simulink library "component_lib"  (R2020b)
settings: Solver=VariableStepAuto  StartTime=0.0  StopTime=10.0  RelTol=1e-3
undefined symbols (not defined in the file or in its folder): ECCV_r, par
libraries: base_lib x70, $bdroot x59, simulink x3, pid_lib x1
(part 2 of 3)

== system component_lib/Thermal Systems ==
  note: TitanX Radiator blockset
  TH0002_radiatorCore : Subsystem  mask{HtH=1.1, StS=0.95, radmodel=52 mm}
      mask prompts: HtH "Effective header to header [m]:"; StS "Effective sideplate to sideplate [m]:"; radmodel "Core depth [m]:"
      mask init:
      | % parameter struct
      | par = struct;
      | 
      | % % get parameters
      | % par.HtH = eval(get_param(gcb, 'HtH'));
      | % par.StS = eval(get_param(gcb, 'StS'));
      | 
      | par.HtH = HtH;
      | par.StS = StS;
      | 
      | % Geometry
      | par.A_face = HtH * StS;
      | 
      | % Total heat transfer coefficient model:
      | par.cUexp = [0.7; 0.8];
      | 
      | switch radmodel
      |     
      |         case '19 mm'
      |         % Core depth
      |         par.CdT = 24e-3;
      |         
      |         % Heat trf. coefficient coefficients
      |         par.cU = [1.118075425066717e-04;
      |                   5.580064095289469e-04;
      |                   2.895685646303412e-05];
      |         
      |         % pressure drop coefficients
      |         par.c_dp_air = [37.253944105671480;
      |                          2.916659649936296e+02];         
      |         par.c_dp_clt = [19.727883408911566;
      |                          5.313528394369467];
      |         
      |         % relative area factors:
      |         rel_air = 0.752767994911226;
      |         rel_clt = 0.127946647958308;
      |     
      |     
      |         case '24 mm'
      |         % Core depth
      |         par.CdT = 24e-3;
      |         
      |         % Heat trf. coefficient coefficients
      |         par.cU = [9.815616404383520e-05;
      |                   4.676700861536502e-04;
      |                   2.415838699598361e-05];
      |         
      |         % pressure drop coefficients
      |         par.c_dp_air = [45.764851256613420;
      |                          2.404056250729179e+02];         
      |         par.c_dp_clt = [18.543378283094310;
      |                          5.151503273505832];
      |         
      |         % relative area factors:
      |         rel_air = 0.733387923444172;
      |         rel_clt = 0.132407142901122;
      |     
      |     
      |     
      |     case '42 mm'
      |         % Core depth
      |         par.CdT = 42e-3;
      |         
      |         % Heat trf. coefficient coefficients
      |         par.cU = [5.544027785616380e-05; 
      |                   2.449228920498670e-04; 
      |                   1.520415888705416e-05];
      |         
      |         % pressure drop coefficients
      |         par.c_dp_air = [36.973761781463810;
      |                          2.758340137219987e+02];
      |         par.c_dp_clt = [19.845956523612838;
      |                          5.112131585795914];
      |         
      |         % relative area factors:
      |         rel_air = 0.752767994911226;
      |         rel_clt = 0.115761252914660;
      |         
      |     case '52 mm'
      |         % Core depth
      |         par.CdT = 52e-3;
      |         
      |         % Heat trf. coefficient coefficients
      |         par.cU = [5.19516413772077e-05;
      |                   0.000198353781023090;
      |                   1.28249375163373e-05];
      |         
      |         % pressure drop coefficients
      |         par.c_dp_air = [46.462548129557995;
      |                          2.255631867184913e+02];
      |         par.c_dp_clt = [18.741626674634468;
      |                          4.871890188700768];
      |         
      |         % relative area factors:
      |         rel_air = 0.7334;
      |         rel_clt = 0.1222;
      | end
      | 
      | 
      | % Flow areas:
      | par.A_air  = rel_air * par.A_face; % Characteristic flow area
      | par.A_clt  = rel_clt * par.CdT * StS;  % Characteristic flow area
      | 
      | % fluid properties
      | setCoolantProperties;
      | setAirProperties;
      mask TypeOptions radmodel: 19 mm | 24 mm | 42 mm | 52 mm
  TH0003_coolantTank : Subsystem  mask{StS=0.95, D_con=0.055, T_0=273 + 25, radmodel=52 mm}
      mask prompts: StS "Sideplate to sideplate [m]"; D_con "Connector internal diameter [m]:"; T_0 "Temperature initial condition [K]:"; radmodel "Core depth [mm]:"
      mask init:
      | par = struct;
      | 
      | % fluid properties
      | setCoolantProperties;
      | setAirProperties;
      | 
      | % pressure drop coeffcient
      | par.zeta = 3;
      | 
      | % set core depth
      | switch radmodel
      |     
      |     case '19 mm'
      |         % Core depth
      |         par.CdT = 19e-3;
      |         
      |     case '24 mm'
      |         % Core depth
      |         par.CdT = 24e-3;
      |     
      |     case '42 mm'
      |         % Core depth
      |         par.CdT = 42e-3;
      |         
      |     case '52 mm'
      |         % Core depth
      |         par.CdT = 52e-3;
      | end
      | 
      | % Geometry
      | % tank volume
      | par.V = par.CdT.^2 * StS;
      | 
      | % inlet area
      | par.A_con = D_con.^2 .* pi/4;
      mask TypeOptions radmodel: 19 mm | 24 mm | 42 mm | 52 mm
  TH0004_radiatorPlugFlow : Subsystem  mask{HtH=1.1, StS=0.95, T_0=286, radmodel=52 mm}
      mask prompts: HtH "Header to header [m]:"; StS "Sideplate to sideplate [m]:"; T_0 "Temperature initial condition [K]:"; radmodel "Core depth [mm]:"
      mask init:
      | par = struct;
      | 
      | % get parameters
      | % par.HtH = eval(get_param(gcb, 'HtH'));
      | % par.StS = eval(get_param(gcb, 'StS'));
      | 
      | par.HtH = HtH;
      | par.StS = StS;
      | 
      | % fluid properties
      | setCoolantProperties;
      | setAirProperties;
      | 
      | 
      | % set core depth
      | switch radmodel
      |     case '42 mm'
      |         % Core depth
      |         par.CdT = 42e-3;
      |         
      |     case '52 mm'
      |         % Core depth
      |         par.CdT = 52e-3;
      | end
      mask TypeOptions radmodel: 19 mm | 24 mm | 42 mm | 52 mm
  TH0005_flowSplit : Subsystem
      mask init:
      | % fluid properties
      | setCoolantProperties;
      | setAirProperties;
  TH0006_flowConfluence : Subsystem  mask{gain=0.01}
      mask prompts: gain "Flow balance gain [-]:"
      mask init:
      | % fluid properties
      | setCoolantProperties;
      | setAirProperties;
  TH0007_airRestriction : Subsystem  mask{A=0.8, zeta=0.3}
      mask prompts: A "Area [m2]:"; zeta "Pressure drop coefficient [-]:"
      mask init:
      | % get parameters
      | % par.A    = eval(get_param(gcb, 'A'));
      | % par.zeta = eval(get_param(gcb, 'zeta'));
      | 
      | par.A    = A;
      | par.zeta = zeta;
      | 
      | % fluid properties
      | setCoolantProperties;
      | setAirProperties;
  TH0008_condenser : Subsystem  mask{HtH=0.85, StS=0.35, cdsmodel=16 mm}
      mask prompts: HtH "Header to header [m]:"; StS "Sideplate to sideplate [m]:"; cdsmodel "Core depth [m]:"
      mask init:
      | % parameter struct
      | par = struct;
      | 
      | % get parameters
      | % par.HtH = eval(get_param(gcb, 'HtH'));
      | % par.StS = eval(get_param(gcb, 'StS'));
      | 
      | par.HtH = HtH;
      | par.StS = StS;
      | 
      | 
      | switch cdsmodel
      |     case '16 mm'
      |         % Core depth
      |         par.CdT = 16-3;
      |         
      |         % pressure drop coefficients
      |         par.c_dp = [2.5; 6];
      |         
      |         
      |     case '18.8 mm'
      |         % Core depth
      |         par.CdT = 18.8e-3;
      |         
      |         % pressure drop coefficients
      |         par.c_dp = [2.7; 11];
      | end
      | 
      | % fluid properties
      | setCoolantProperties;
      | setAirProperties;
      mask TypeOptions cdsmodel: 16 mm | 18.8 mm
  TH0009_intake : Subsystem  mask{zeta=0.9}
      mask prompts: zeta "Pressure increase coefficient [-]:"
      mask init:
      | % get parameters
      | % par.zeta = eval(get_param(gcb, 'zeta'));
      | par.zeta = zeta;
      | 
      | % fluid properties
      | setCoolantProperties;
      | setAirProperties;
  TH0010_fan : Subsystem  mask{n_fan=4}
      mask prompts: n_fan "Nr. of fans [-]:"
      mask init:
      | % parameter struct
      | par = struct;
      | 
      | % get parameters
      | % par.n_fan = eval(get_param(gcb, 'n_fan'));
      | par.n_fan = n_fan;
      | 
      | 
      | % fan parameters
      | par.dpr   = -200;
      | par.q0    = 4290/3600;
      | par.dp0   = 800;
      | par.P_nom = 832;
      | 
      | 
      | % fluid properties
      | setCoolantProperties;
      | setAirProperties;
  TH0011_coolingChannel : Subsystem  mask{d=2e-3, L=50e-2, n_ch=1}
      mask prompts: d "Hydraulic diameter [m]:"; L "Length [m]:"; n_ch "Nr. of channels [-]:"
      mask init:
      | % parameter struct
      | par = struct;
      | par.d = d;
      | par.L = L;
      | 
      | % fluid properties
      | setCoolantProperties;
      | setAirProperties;
  TH0011_outletFlowBalance : Subsystem  mask{gain=0.05}
      mask prompts: gain "Dyn. balancing factor [m]:"
      mask init:
      | % fluid properties
      | setCoolantProperties;
      | setAirProperties;
  TH0011_pipe : Subsystem  mask{d=5e-2, L=1, T_0=273 + 20, p_0=2e5, W_0=2}
      mask prompts: d "Diameter [m]:"; L "Length [m]:"; T_0 "Initial temperature [K]:"; p_0 "Initial pressure [Pa]:"; W_0 "Initial flow [kg/s]:"
      mask init:
      | % parameter struct
      | par = struct;
      | 
      | % get parameters
      | % par.d = eval(get_param(gcb, 'd'));
      | % par.L = eval(get_param(gcb, 'L'));
      | 
      | par.d = d;
      | par.L = L;
      | 
      | % fluid properties
      | setCoolantProperties;
      | setAirProperties;
  TH0011_thermalMass : Subsystem  mask{m=34, cp=691, T_0=273 + 20}
      mask prompts: m "Mass [kg]:"; cp "Heat capacity [J/kgK]:"; T_0 "Initial temperature [K]:"
      mask init:
      | % fluid properties
      | setCoolantProperties;
      | setAirProperties;
  TH0012_equalSplitMerge : Subsystem  mask{n=1}
      mask prompts: n "Split/merge flow [-]"
      mask init:
      | % fluid properties
      | setCoolantProperties;
      | setAirProperties;
  TH0013_tank : Subsystem  mask{V=5e-3}
      mask prompts: V "Volume [m3]:"
      mask init:
      | % fluid properties
      | setCoolantProperties;
      | setAirProperties;
  TH0014_valve : Subsystem  mask{d=10e-2, dr=5e-2, C_d=0.9}
      mask prompts: d "Inlet port diameter [m]:"; dr "Restriction diameter [m]:"; C_d "Discharge coefficient [-]:"
      mask init:
      | % parameter struct
      | par = struct;
      | 
      | % get parameters
      | % par.d    = eval(get_param(gcb, 'd'));
      | % par.dr   = eval(get_param(gcb, 'dr'));
      | % par.C_d  = eval(get_param(gcb, 'C_d'));
      | 
      | par.d    = d;
      | par.dr   = dr;
      | par.C_d  = C_d;
      | 
      | 
      | % fluid properties
      | setCoolantProperties;
      | setAirProperties;
  TH0015_totalHeatTransfer : Subsystem
      mask init:
      | % parameter struct
      | par = struct;
      | 
      | % fluid properties
      | setCoolantProperties;
      | setAirProperties;

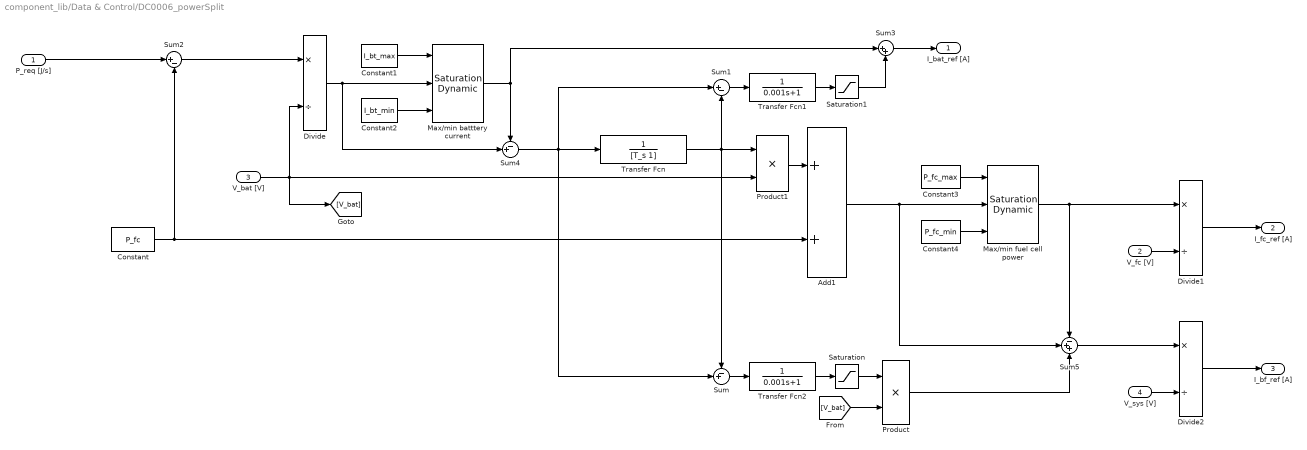
== system component_lib/Data & Control/DC0006_powerSplit ==
  P_req [J/s] : Inport
  V_fc [V] : Inport  Port=2
  V_bat [V] : Inport  Port=3
  V_sys [V] : Inport  Port=4
  Add1 : Sum
  Constant : Constant  Value=P_fc
  Constant1 : Constant  Value=I_bt_max
  Constant2 : Constant  Value=I_bt_min
  Constant3 : Constant  Value=P_fc_max
  Constant4 : Constant  Value=P_fc_min
  Divide : Product  Inputs=*/
  Divide1 : Product  Inputs=*/
  Divide2 : Product  Inputs=*/
  Max/min batttery current : simulink/Discontinuities/Saturation Dynamic  OutMin=[]  OutMax=[]  OutDataTypeStr=Inherit: Same as second input  OutDataType=fixdt(1, 16)  OutScaling=2^-10  DoSatur=off
  Max/min fuel cell power : simulink/Discontinuities/Saturation Dynamic  OutMin=[]  OutMax=[]  OutDataTypeStr=Inherit: Same as second input  OutDataType=fixdt(1, 16)  OutScaling=2^-10  DoSatur=off
  Product : Product
  Product1 : Product
  Saturation : Saturate  UpperLimit=0  LowerLimit=-inf
  Saturation1 : Saturate  UpperLimit=inf  LowerLimit=0
  Sum : Sum  Inputs=-+|
  Sum1 : Sum  Inputs=|+-
  Sum2 : Sum  Inputs=|+-
  Sum3 : Sum  Inputs=|++
  Sum4 : Sum  Inputs=-+|
  Sum5 : Sum  Inputs=-++
  Transfer Fcn : TransferFcn  Denominator=[T_s 1]
  Transfer Fcn1 : TransferFcn  Denominator=[0.001 1]
  Transfer Fcn2 : TransferFcn  Denominator=[0.001 1]
  I_bat_ref [A] : Outport
  I_fc_ref [A] : Outport  Port=2
  I_bf_ref [A] : Outport  Port=3
  wires:
  Sum2/1 -> Divide/1
  Divide1/1 -> I_fc_ref [A]/1
  V_bat [V]/1 -> Product1/2, [V_bat], Divide/2
  Constant/1 -> Sum2/2, Add1/2
  Divide/1 -> Max/min batttery current/2, Sum4/2
  Constant1/1 -> Max/min batttery current/1
  Constant2/1 -> Max/min batttery current/3
  Add1/1 -> Sum5/2, Max/min fuel cell power/2
  Constant3/1 -> Max/min fuel cell power/1
  Constant4/1 -> Max/min fuel cell power/3
  Max/min fuel cell power/1 -> Sum5/1, Divide1/1
  Sum5/1 -> Divide2/1
  V_sys [V]/1 -> Divide2/2
  Divide2/1 -> I_bf_ref [A]/1
  V_fc [V]/1 -> Divide1/2
  Product1/1 -> Add1/1
  P_req [J/s]/1 -> Sum2/1
  Max/min batttery current/1 -> Sum3/1, Sum4/1
  Sum4/1 -> Sum1/1, Sum/2, Transfer Fcn/1
  Transfer Fcn/1 -> Sum1/2, Product1/1, Sum/1
  [V_bat] -> Product/2
  Saturation/1 -> Product/1
  Product/1 -> Sum5/3
  Saturation1/1 -> Sum3/2
  Sum3/1 -> I_bat_ref [A]/1
  Sum1/1 -> Transfer Fcn1/1
  Transfer Fcn1/1 -> Saturation1/1
  Sum/1 -> Transfer Fcn2/1
  Transfer Fcn2/1 -> Saturation/1

== system component_lib/Data & Control/DC0007_cathodeFlowControl ==
  note: Oxygen flow [kg/s]
  note: Reference oxygen flow [kg/s]
  I_fc [A] : Inport
  W_ca [kg/s] : Inport  Port=2
  Cells in FC stack : Constant  Value=n_cell
  F0003_reactionFlow.m : base_lib/F0003_pukrushpan2004/F0003_reactionFlow.m  SystemSampleTime=-1  VariantActivationTime=update diagram  Latency=0  AutoFrameSizeCalculation=off
  Gain : Gain  Gain=1e5
  Gain1 : Gain  Gain=-1
  Oxygen mass fraction in dry air : Constant  Value=0.23
  Oxygen stoichiometry reference : Constant  Value=lambda_O2_ref
  PID Controller : pid_lib/PID Controller  Controller=PID  Form=Parallel  TimeDomain=Continuous-time  UseExternalTs=off  SampleTime=-1  IntegratorMethod=Forward Euler  FilterMethod=Forward Euler  ControllerParametersSource=internal  P=1  I=1  D=0  UseFilter=on  N=100  TunerSelectOption=Transfer Function Based (PID Tuner App)  InitialConditionSource=internal  InitialConditionForIntegrator=0  InitialConditionForFilter=0  DifferentiatorICPrevScaledInput=0  ExternalReset=none  TrackingMode=off  Kt=1  LimitOutput=on  SatLimitsSource=internal  UpperSaturationLimit=2e4  LowerSaturationLimit=3e3  LinearizeAsGain=on  AntiWindupMode=back-calculation  Kb=1e-1  POutMin=[]  POutMax=[]  IOutMin=[]  IOutMax=[]  DOutMin=[]  DOutMax=[]  NOutMin=[]  NOutMax=[]  SumOutMin=[]  SumOutMax=[]  SaturationOutMin=[]  SaturationOutMax=[]  PParamMin=[]  PParamMax=[]  IParamMin=[]  IParamMax=[]  DParamMin=[]  DParamMax=[]  NParamMin=[]  NParamMax=[]  KbParamMin=[]  KbParamMax=[]  KtParamMin=[]  KtParamMax=[]  KbOutMin=[]  KbOutMax=[]  KtOutMin=[]  KtOutMax=[]  IntegratorOutMin=[]  IntegratorOutMax=[]  FilterOutMin=[]  FilterOutMax=[]  SumI1OutMin=[]  SumI1OutMax=[]  SumI2OutMin=[]  SumI2OutMax=[]  SumI3OutMin=[]  SumI3OutMax=[]  SumI4OutMin=[]  SumI4OutMax=[]  SumDOutMin=[]  SumDOutMax=[]  DifferentiatorOutMin=[]  DifferentiatorOutMax=[]  FilterDiffOutCoefMin=[]  FilterDiffOutCoefMax=[]  ReciprocalOutMin=[]  ReciprocalOutMax=[]  SumDenOutMin=[]  SumDenOutMax=[]  SumNumOutMin=[]  SumNumOutMax=[]  DivideOutMin=[]  DivideOutMax=[]  UdiffTsProdOutMin=[]  UdiffTsProdOutMax=[]  NTsProdOutMin=[]  NTsProdOutMax=[]  UintegralTsProdOutMin=[]  UintegralTsProdOutMax=[]  UngainTsProdOutMin=[]  UngainTsProdOutMax=[]  IntegratorContinuousStateAttributes=''  IntegratorStateMustResolveToSignalObject=off  IntegratorRTWStateStorageClass=Auto  FilterContinuousStateAttributes=''  FilterStateMustResolveToSignalObject=off  FilterRTWStateStorageClass=Auto  ParallelPVariant=InternalParameters  IdealPVariant=Disabled  IVariant=InternalParameters  DVariant=InternalParameters  IntegratorVariant=Continuous  SatVariant=Enabled  AWVariant=BackCalculation  PCopyVariant=Disabled  TRVariant=Disabled  FdbkBlocksVariant=Forward  IdealPFdbkVariant=Disabled  SatFdbkVariant=Disabled  DerivativeFilterVariant=ContFilter  NVariant=InternalParameters  NCopyVariant=Disabled  FilterICVariant=InternalICsFilter  IntegratorICVariant=InternalICs  ExternalResetVariant=Disabled  TRSumVariant=Passthrough  SumFdbkVariant=Disabled  SumVariant=Sum_PID  TsampFilterVariant=InternalTs  TsampNgainVariant=Passthrough  TsampIntegralVariant=Passthrough  ExternalSaturationOutDataTypeStr=Inherit: Same as second input
  Product : Product  Inputs=3
  Product1 : Product
  Selector : Selector  InputPortWidth=4  IndexOptions=Index vector (dialog)  Indices=2  OutputSizes=1
  Sum : Sum  Inputs=|+-
  Terminator : Terminator
  w_cmp [rad/s] : Outport
  wires:
  F0003_reactionFlow.m/2 -> Selector/1
  Oxygen stoichiometry reference/1 -> Product/1
  Selector/1 -> Gain1/1
  Oxygen mass fraction in dry air/1 -> Product1/2
  F0003_reactionFlow.m/1 -> Terminator/1
  Gain1/1 -> Product/3
  Cells in FC stack/1 -> Product/2
  Product/1 -> Sum/1
  Product1/1 -> Sum/2
  Sum/1 -> Gain/1
  PID Controller/1 -> w_cmp [rad/s]/1
  Gain/1 -> PID Controller/1
  I_fc [A]/1 -> F0003_reactionFlow.m/1
  W_ca [kg/s]/1 -> Product1/1

== system component_lib/Data & Control/DC0010_anodeTankFlowControl ==
  note: Flow feedback - adjust +- 50%
  note: Flow feed-forward
  p [Pa] : Inport
  I_fc [A] : Inport  Port=2
  p_ref [Pa] : Inport  Port=3
  Cells in FC stack : Constant  Value=n_cell
  F0003_reactionFlow.m : base_lib/F0003_pukrushpan2004/F0003_reactionFlow.m  SystemSampleTime=-1  VariantActivationTime=update diagram  Latency=0  AutoFrameSizeCalculation=off
  Gain : Gain  Gain=1e-6
  Gain1 : Gain  Gain=-1
  Product : Product
  Product1 : Product
  Saturation : Saturate
  Selector : Selector  InputPortWidth=4  IndexOptions=Index vector (dialog)  Indices=1  OutputSizes=1
  Sum : Sum  Inputs=|+-
  Sum1 : Sum  Inputs=|++
  Terminator : Terminator
  W_H2_tank [kg/s] : Outport
  wires:
  Gain1/1 -> Product/2
  Selector/1 -> Gain1/1
  F0003_reactionFlow.m/1 -> Selector/1
  I_fc [A]/1 -> F0003_reactionFlow.m/1
  F0003_reactionFlow.m/2 -> Terminator/1
  Cells in FC stack/1 -> Product/1
  p_ref [Pa]/1 -> Sum/1
  p [Pa]/1 -> Sum/2
  Product/1 -> Sum1/1, Product1/1
  Sum1/1 -> W_H2_tank [kg/s]/1
  Sum/1 -> Gain/1
  Product1/1 -> Sum1/2
  Gain/1 -> Saturation/1
  Saturation/1 -> Product1/2

== system component_lib/Data & Control/SC0002_signalRead ==
  SigIdentifier : Inport
  tag scope: SigIdentifier=global
  wires:
  SigIdentifier/1 -> [SigIdentifier]

== system component_lib/Data & Control/SC0003_signalWrite ==
  y : Outport
  wires:
  [SigIdentifier] -> y/1

== system component_lib/Electrochemistry/EL0001_panasonicNCR18650PF ==
  note: Kelvin -> degC
  note: Power Loss
  I [A] : Inport
  T [K] : Inport  Port=2
  Abs : Abs
  Constant : Constant  Value=273.15
  Constant5 : Constant  Value=3.6e3
  Divide1 : Product  Inputs=*//
  F0001_cellCapacity.m : base_lib/F0001_panasonicCell/F0001_cellCapacity.m  SystemSampleTime=-1  VariantActivationTime=update diagram  Latency=0  AutoFrameSizeCalculation=off
      settings: SourceProductBaseCode=SL
  F0001_dynamicVoltage.m : base_lib/F0001_panasonicCell/F0001_dynamicVoltage.m  SystemSampleTime=-1  VariantActivationTime=update diagram  Latency=0  AutoFrameSizeCalculation=off
  F0001_ocvSOC.m : base_lib/F0001_panasonicCell/F0001_ocvSOC.m  SystemSampleTime=-1  VariantActivationTime=update diagram  Latency=0  AutoFrameSizeCalculation=off
      settings: SourceProductBaseCode=SL
  Gain : Gain  Gain=-1
  Integrator Limited : Integrator  InitialCondition=par.init_SOC  LimitOutput=on  UpperSaturationLimit=1  LowerSaturationLimit=0
  Integrator1 : Integrator  InitialCondition=zeros(5,1)
  Product : Product
  Product2 : Product
  Saturation : Saturate  UpperLimit=0.9  LowerLimit=0.1
  Sum : Sum  Inputs=|+-
  Sum1 : Sum  Inputs=+|-
  Sum2 : Sum  Inputs=|+-
  V [V] : Outport
  SOC [-] : Outport  Port=2
  Q_gen [J/s] : Outport  Port=3
  wires:
  F0001_dynamicVoltage.m/1 -> Integrator1/1
  Integrator1/1 -> F0001_dynamicVoltage.m/1
  T [K]/1 -> Sum2/1
  F0001_ocvSOC.m/1 -> Product/1, Sum/1
  Integrator Limited/1 -> SOC [-]/1, Saturation/1
  Sum/1 -> V [V]/1, Product2/2
  I [A]/1 -> F0001_dynamicVoltage.m/3, Gain/1, [i]
  Product/1 -> Sum1/1
  Product2/1 -> Sum1/2
  Sum1/1 -> Abs/1
  Abs/1 -> Q_gen [J/s]/1
  Constant/1 -> Sum2/2
  Sum2/1 -> F0001_dynamicVoltage.m/2, F0001_cellCapacity.m/1
  Constant5/1 -> Divide1/2
  F0001_cellCapacity.m/1 -> Divide1/3
  Gain/1 -> Divide1/1
  Divide1/1 -> Integrator Limited/1
  F0001_dynamicVoltage.m/2 -> Sum/2
  [i] -> Product2/1, Product/2
  Saturation/1 -> F0001_ocvSOC.m/1

== system component_lib/Electrochemistry/EL0003_pCell ==
  I [A] : Inport
  T [K] : Inport  Port=2
  F0002_pStackVoltage.m : base_lib/F0002_pStack/F0002_pStackVoltage.m  SystemSampleTime=-1  VariantActivationTime=update diagram  Latency=0  AutoFrameSizeCalculation=off
  F0003_reactionFlow.m : base_lib/F0003_pukrushpan2004/F0003_reactionFlow.m  SystemSampleTime=-1  VariantActivationTime=update diagram  Latency=0  AutoFrameSizeCalculation=off
  V [V] : Outport
  Q_gen [J/s] : Outport  Port=2
  W_an [kg/s] : Outport  Port=3
  W_ca [kg/s] : Outport  Port=4
  wires:
  I [A]/1 -> F0003_reactionFlow.m/1, F0002_pStackVoltage.m/1
  F0002_pStackVoltage.m/1 -> V [V]/1
  T [K]/1 -> F0002_pStackVoltage.m/2
  F0002_pStackVoltage.m/2 -> Q_gen [J/s]/1
  F0003_reactionFlow.m/1 -> W_an [kg/s]/1
  F0003_reactionFlow.m/2 -> W_ca [kg/s]/1

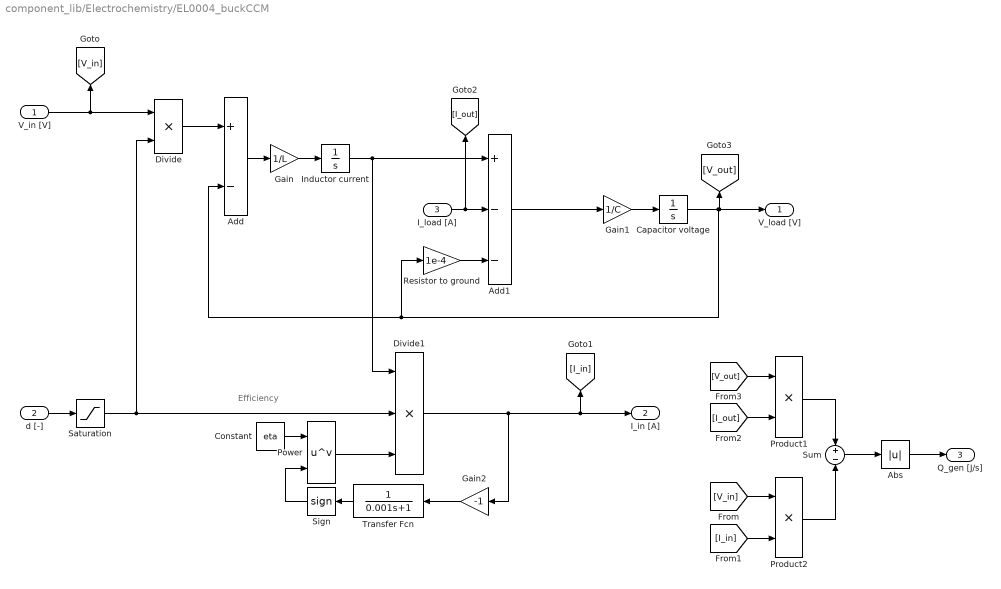
== system component_lib/Electrochemistry/EL0004_buckCCM ==
  note: Efficiency
  V_in [V] : Inport
  d [-] : Inport  Port=2
  I_load [A] : Inport  Port=3
  Abs : Abs
  Add : Sum  Inputs=+-
  Add1 : Sum  Inputs=+--
  Capacitor voltage : Integrator  InitialCondition=V_init
  Constant : Constant  Value=eta
  Divide : Product  Inputs=**
  Divide1 : Product  Inputs=***
  Gain : Gain  Gain=1/L
  Gain1 : Gain  Gain=1/C
  Gain2 : Gain  Gain=-1
  Inductor current : Integrator
  Power : Math  Operator=pow  SaturateOnIntegerOverflow=on
  Product1 : Product
  Product2 : Product
  "Resistor to ground " : Gain  Gain=1e-4
  Saturation : Saturate  UpperLimit=1  LowerLimit=0
  Sign : Signum
  Sum : Sum  Inputs=+|-
  Transfer Fcn : TransferFcn  Denominator=[0.001 1]
  V_load [V] : Outport
  I_in [A] : Outport  Port=2
  Q_gen [J/s] : Outport  Port=3
  wires:
  Divide1/1 -> Gain2/1, I_in [A]/1, [I_in]
  Abs/1 -> Q_gen [J/s]/1
  Sum/1 -> Abs/1
  Product2/1 -> Sum/2
  Product1/1 -> Sum/1
  [V_out] -> Product1/1
  [I_out] -> Product1/2
  [I_in] -> Product2/2
  [V_in] -> Product2/1
  Gain2/1 -> Transfer Fcn/1
  Transfer Fcn/1 -> Sign/1
  Constant/1 -> Power/1
  Power/1 -> Divide1/3
  Sign/1 -> Power/2
  "Resistor to ground "/1 -> Add1/3
  d [-]/1 -> Saturation/1
  V_in [V]/1 -> [V_in], Divide/1
  I_load [A]/1 -> [I_out], Add1/2
  Gain1/1 -> Capacitor voltage/1
  Add1/1 -> Gain1/1
  Inductor current/1 -> Add1/1, Divide1/1
  Gain/1 -> Inductor current/1
  Capacitor voltage/1 -> [V_out], V_load [V]/1, Add/2, "Resistor to ground "/1
  Saturation/1 -> Divide/2, Divide1/2
  Add/1 -> Gain/1
  Divide/1 -> Add/1

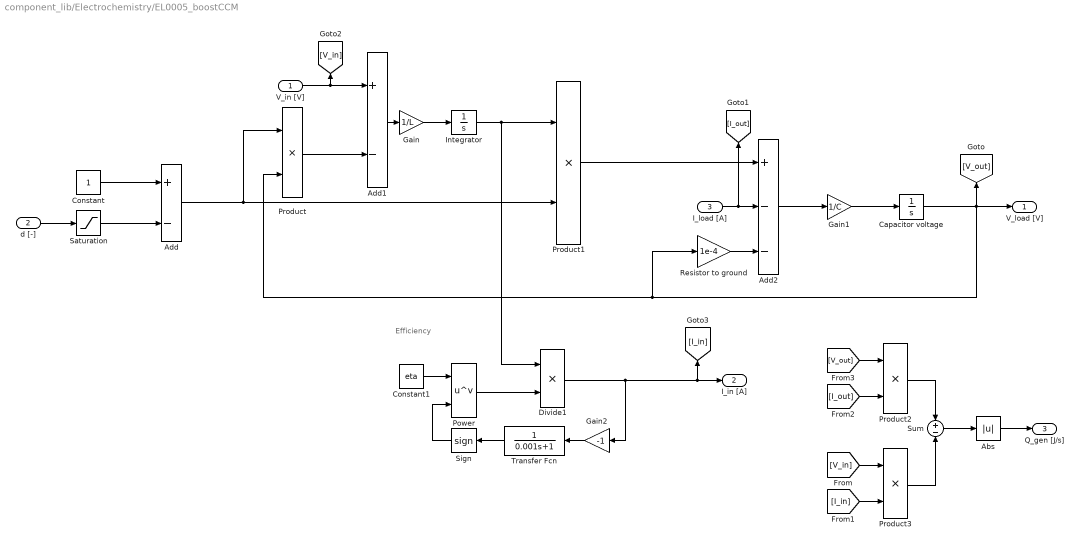
== system component_lib/Electrochemistry/EL0005_boostCCM ==
  note: Efficiency
  V_in [V] : Inport
  d [-] : Inport  Port=2
  I_load [A] : Inport  Port=3
  Abs : Abs
  Add : Sum  Inputs=+-
  Add1 : Sum  Inputs=+-
  Add2 : Sum  Inputs=+--
  Capacitor voltage : Integrator  InitialCondition=V_init
  Constant : Constant
  Constant1 : Constant  Value=eta
  Divide1 : Product  Inputs=**
  Gain : Gain  Gain=1/L
  Gain1 : Gain  Gain=1/C
  Gain2 : Gain  Gain=-1
  Integrator : Integrator
  Power : Math  Operator=pow  SaturateOnIntegerOverflow=on
  Product{,1..3} (4 alike) : Product
  Resistor to ground : Gain  Gain=1e-4
  Saturation : Saturate  UpperLimit=0.8  LowerLimit=0.2
  Sign : Signum
  Sum : Sum  Inputs=+|-
  Transfer Fcn : TransferFcn  Denominator=[0.001 1]
  V_load [V] : Outport
  I_in [A] : Outport  Port=2
  Q_gen [J/s] : Outport  Port=3
  wires:
  Divide1/1 -> I_in [A]/1, [I_in], Gain2/1
  Abs/1 -> Q_gen [J/s]/1
  Sum/1 -> Abs/1
  [V_out] -> Product2/1
  [V_in] -> Product3/1
  [I_out] -> Product2/2
  [I_in] -> Product3/2
  Product2/1 -> Sum/1
  Product3/1 -> Sum/2
  Power/1 -> Divide1/2
  Transfer Fcn/1 -> Sign/1
  Gain2/1 -> Transfer Fcn/1
  Sign/1 -> Power/2
  Constant1/1 -> Power/1
  Resistor to ground/1 -> Add2/3
  V_in [V]/1 -> Add1/1, [V_in]
  d [-]/1 -> Saturation/1
  I_load [A]/1 -> Add2/2, [I_out]
  Gain1/1 -> Capacitor voltage/1
  Add2/1 -> Gain1/1
  Product1/1 -> Add2/1
  Integrator/1 -> Product1/1, Divide1/1
  Add1/1 -> Gain/1
  Product/1 -> Add1/2
  Add/1 -> Product1/2, Product/1
  Gain/1 -> Integrator/1
  Capacitor voltage/1 -> V_load [V]/1, [V_out], Product/2, Resistor to ground/1
  Constant/1 -> Add/1
  Saturation/1 -> Add/2

== system component_lib/Electrochemistry/EL0006_parallelVoltageSources ==
  V_1 [V] : Inport
  I_load [A] : Inport  Port=2
  V_2 [V] : Inport  Port=3
  Divide : Product  Inputs=*/
  Divide1 : Product  Inputs=*/
  Gain : Gain  Gain=1/C
  Gain1 : Gain  Gain=1e-3
  R : Constant  Value=R
  Sum : Sum  Inputs=|+-
  Sum1 : Sum  Inputs=-+|
  Sum2 : Sum  Inputs=|+-
  Sum3 : Sum  Inputs=+-+
  V_4 : Integrator  InitialCondition=V_init
  I_1 [A] : Outport
  V_3 [V] : Outport  Port=2
  I_2 [A] : Outport  Port=3
  wires:
  Gain1/1 -> Sum/2
  Sum/1 -> Gain/1
  Sum3/1 -> Sum/1
  V_4/1 -> Sum1/1, Gain1/1, Sum2/2, V_3 [V]/1
  Divide1/1 -> Sum3/3, I_2 [A]/1
  V_1 [V]/1 -> Sum1/2
  I_load [A]/1 -> Sum3/2
  Gain/1 -> V_4/1
  Divide/1 -> Sum3/1, I_1 [A]/1
  V_2 [V]/1 -> Sum2/1
  Sum2/1 -> Divide1/1
  R/1 -> Divide/2, Divide1/2
  Sum1/1 -> Divide/1

== system component_lib/Gas Exchange/GE0001_humidGasSupply ==
  Constant : Constant  Value=par.p_tot
  Constant1 : Constant  Value=par.RH
  Constant2 : Constant  Value=par.T
  Constant3 : Constant  Value=par.x_H2
  Constant4 : Constant  Value=par.x_O2
  F0010_pressureSupply.m : base_lib/F0010_gasFlow/F0010_pressureSupply.m  SystemSampleTime=-1  VariantActivationTime=update diagram  Latency=0  AutoFrameSizeCalculation=off
  F0010_vaporSaturationPressure.m : base_lib/F0010_gasFlow/F0010_vaporSaturationPressure.m  SystemSampleTime=-1  VariantActivationTime=update diagram  Latency=0  AutoFrameSizeCalculation=off
  p (p x 4) : Outport
  T [K] : Outport  Port=2
  wires:
  Constant2/1 -> T [K]/1, F0010_vaporSaturationPressure.m/1
  Constant/1 -> F0010_pressureSupply.m/1
  F0010_vaporSaturationPressure.m/1 -> F0010_pressureSupply.m/5
  Constant1/1 -> F0010_pressureSupply.m/4
  Constant3/1 -> F0010_pressureSupply.m/2
  Constant4/1 -> F0010_pressureSupply.m/3
  F0010_pressureSupply.m/1 -> p (p x 4)/1

== system component_lib/Gas Exchange/GE0002_dynHumidGasSupply ==
  T [K] : Inport
  p_ref [Pa] : Inport  Port=2
  RH [-] : Inport  Port=3
  Constant : Constant  Value=x_H2_dry
  Constant1 : Constant  Value=x_O2_dry
  F0010_pressureSupply.m : base_lib/F0010_gasFlow/F0010_pressureSupply.m  SystemSampleTime=-1  VariantActivationTime=update diagram  Latency=0  AutoFrameSizeCalculation=off
      settings: SourceProductBaseCode=SL
  F0010_vaporSaturationPressure.m : base_lib/F0010_gasFlow/F0010_vaporSaturationPressure.m  SystemSampleTime=-1  VariantActivationTime=update diagram  Latency=0  AutoFrameSizeCalculation=off
      settings: SourceProductBaseCode=SL
  p (p x 4) : Outport
  T_out [K] : Outport  Port=2
  wires:
  p_ref [Pa]/1 -> F0010_pressureSupply.m/1
  T [K]/1 -> F0010_vaporSaturationPressure.m/1, T_out [K]/1
  F0010_vaporSaturationPressure.m/1 -> F0010_pressureSupply.m/5
  RH [-]/1 -> F0010_pressureSupply.m/4
  F0010_pressureSupply.m/1 -> p (p x 4)/1
  Constant/1 -> F0010_pressureSupply.m/2
  Constant1/1 -> F0010_pressureSupply.m/3

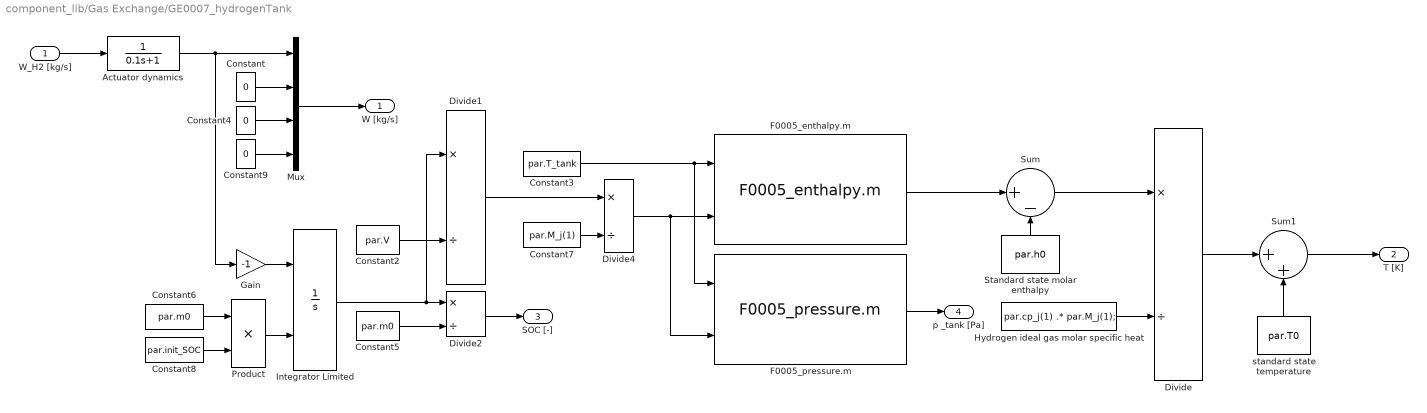
== system component_lib/Gas Exchange/GE0007_hydrogenTank ==
  W_H2 [kg/s] : Inport
  Actuator dynamics : TransferFcn  Denominator=[0.1 1]
  Constant : Constant  Value=0
  Constant2 : Constant  Value=par.V
  Constant3 : Constant  Value=par.T_tank
  Constant4 : Constant  Value=0
  Constant5 : Constant  Value=par.m0
  Constant6 : Constant  Value=par.m0
  Constant7 : Constant  Value=par.M_j(1)
  Constant8 : Constant  Value=par.init_SOC
  Constant9 : Constant  Value=0
  Divide{,1..2,4} (4 alike) : Product  Inputs=*/
  F0005_enthalpy.m : base_lib/F0005_h2Thermodynamics/F0005_enthalpy.m  SystemSampleTime=-1  VariantActivationTime=update diagram  Latency=0  AutoFrameSizeCalculation=off
  F0005_pressure.m : base_lib/F0005_h2Thermodynamics/F0005_pressure.m  SystemSampleTime=-1  VariantActivationTime=update diagram  Latency=0  AutoFrameSizeCalculation=off
  Gain : Gain  Gain=-1
  Hydrogen ideal gas molar specific heat : Constant  Value=par.cp_j(1) .* par.M_j(1);
  Integrator Limited : Integrator  InitialConditionSource=external  LimitOutput=on  LowerSaturationLimit=0
  Mux : Mux
  Product : Product
  Standard state molar enthalpy : Constant  Value=par.h0
  Sum : Sum  Inputs=|+-
  Sum1 : Sum  Inputs=|++
  standard state temperature : Constant  Value=par.T0
  W [kg/s] : Outport
  T [K] : Outport  Port=2
  SOC [-] : Outport  Port=3
  p _tank [Pa] : Outport  Port=4
  wires:
  Integrator Limited/1 -> Divide1/1, Divide2/1
  Constant2/1 -> Divide1/2
  Constant3/1 -> F0005_pressure.m/1, F0005_enthalpy.m/1
  F0005_pressure.m/1 -> p _tank [Pa]/1
  Divide2/1 -> SOC [-]/1
  Hydrogen ideal gas molar specific heat/1 -> Divide/2
  Divide1/1 -> Divide4/1
  Constant7/1 -> Divide4/2
  Divide4/1 -> F0005_enthalpy.m/2, F0005_pressure.m/2
  F0005_enthalpy.m/1 -> Sum/1
  Standard state molar enthalpy/1 -> Sum/2
  Sum/1 -> Divide/1
  Divide/1 -> Sum1/1
  standard state temperature/1 -> Sum1/2
  Sum1/1 -> T [K]/1
  Constant5/1 -> Divide2/2
  Constant6/1 -> Product/1
  Product/1 -> Integrator Limited/2
  Constant8/1 -> Product/2
  Constant9/1 -> Mux/4
  Constant/1 -> Mux/2
  Constant4/1 -> Mux/3
  Actuator dynamics/1 -> Gain/1, Mux/1
  Mux/1 -> W [kg/s]/1
  Gain/1 -> Integrator Limited/1
  W_H2 [kg/s]/1 -> Actuator dynamics/1

== system component_lib/Gas Exchange/GE0008_gasProperties ==
  p (p x 4) : Inport
  T [K] : Inport  Port=2
  Demux : Demux
  Divide : Product  Inputs=*/
  F0010_vaporSaturationPressure.m : base_lib/F0010_gasFlow/F0010_vaporSaturationPressure.m  SystemSampleTime=-1  VariantActivationTime=update diagram  Latency=0  AutoFrameSizeCalculation=off
      settings: SourceProductBaseCode=SL
  Mux : Mux
  Sum : Sum  Inputs=|+|
  p [Pa] : Outport
  RH [-] : Outport  Port=2
  wires:
  Sum/1 -> p [Pa]/1
  p (p x 4)/1 -> Demux/1
  Demux/1 -> Mux/1
  Demux/2 -> Mux/2
  Demux/3 -> Divide/1, Mux/3
  Demux/4 -> Mux/4
  Mux/1 -> Sum/1
  Divide/1 -> RH [-]/1
  F0010_vaporSaturationPressure.m/1 -> Divide/2
  T [K]/1 -> F0010_vaporSaturationPressure.m/1

== system component_lib/Gas Exchange/GE0009_controlVolume ==
  note: Pressure
  note: Mass flow contribution
      | to pressure dynamics
  dW (W,W,W,W) : Inport
  T_1 [K] : Inport  Port=2
  Constant : Constant  Value=par.p0
  Constant1 : Constant  Value=par.RH0
  Constant2 : Constant  Value=par.T0
  Constant3 : Constant  Value=par.V
  Constant5 : Constant  Value=par.x0_H2
  Constant6 : Constant  Value=par.x0_O2
  Divide1 : Product  Inputs=***/
  F0010_pressureSupply.m : base_lib/F0010_gasFlow/F0010_pressureSupply.m  SystemSampleTime=-1  VariantActivationTime=update diagram  Latency=0  AutoFrameSizeCalculation=off
      settings: SourceProductBaseCode=SL
  F0010_vaporSaturationPressure.m : base_lib/F0010_gasFlow/F0010_vaporSaturationPressure.m  SystemSampleTime=-1  VariantActivationTime=update diagram  Latency=0  AutoFrameSizeCalculation=off
      settings: SourceProductBaseCode=SL
  Gas constants : Constant  Value=par.R_j
  Integrator Limited1 : Integrator  InitialConditionSource=external  LimitOutput=on  LowerSaturationLimit=10
  p (p,p,p,p) : Outport
  T_2 [K] : Outport  Port=2
  wires:
  Integrator Limited1/1 -> p (p,p,p,p)/1
  T_1 [K]/1 -> T_2 [K]/1, Divide1/3
  Constant/1 -> F0010_pressureSupply.m/1
  F0010_pressureSupply.m/1 -> Integrator Limited1/2
  dW (W,W,W,W)/1 -> Divide1/1
  Divide1/1 -> Integrator Limited1/1
  Constant3/1 -> Divide1/4
  Gas constants/1 -> Divide1/2
  F0010_vaporSaturationPressure.m/1 -> F0010_pressureSupply.m/5
  Constant1/1 -> F0010_pressureSupply.m/4
  Constant5/1 -> F0010_pressureSupply.m/2
  Constant6/1 -> F0010_pressureSupply.m/3
  Constant2/1 -> F0010_vaporSaturationPressure.m/1

== system component_lib/Gas Exchange/GE0010_flowRestriction ==
  p_1 (p,p,p,p) : Inport
  T_1 [K] : Inport  Port=2
  p_2 (p,p,p,p) : Inport  Port=3
  T_2 [K] : Inport  Port=4
  Constant : Constant
  F0010_compressibleRestriction.m : base_lib/F0010_gasFlow/F0010_compressibleRestriction.m  SystemSampleTime=-1  VariantActivationTime=update diagram  Latency=0  AutoFrameSizeCalculation=off
      settings: SourceProductBaseCode=SL
  Ground : Ground
  W (W,W,W,W) : Outport
  T_out [K] : Outport  Port=2
  "[--]" : Outport  Port=3
  "[---]" : Outport  Port=4
  wires:
  p_1 (p,p,p,p)/1 -> F0010_compressibleRestriction.m/1
  p_2 (p,p,p,p)/1 -> F0010_compressibleRestriction.m/2
  T_1 [K]/1 -> T_out [K]/1, F0010_compressibleRestriction.m/3
  Ground/1 -> "[--]"/1, "[---]"/1
  F0010_compressibleRestriction.m/1 -> W (W,W,W,W)/1
  T_2 [K]/1 -> F0010_compressibleRestriction.m/4
  Constant/1 -> F0010_compressibleRestriction.m/5

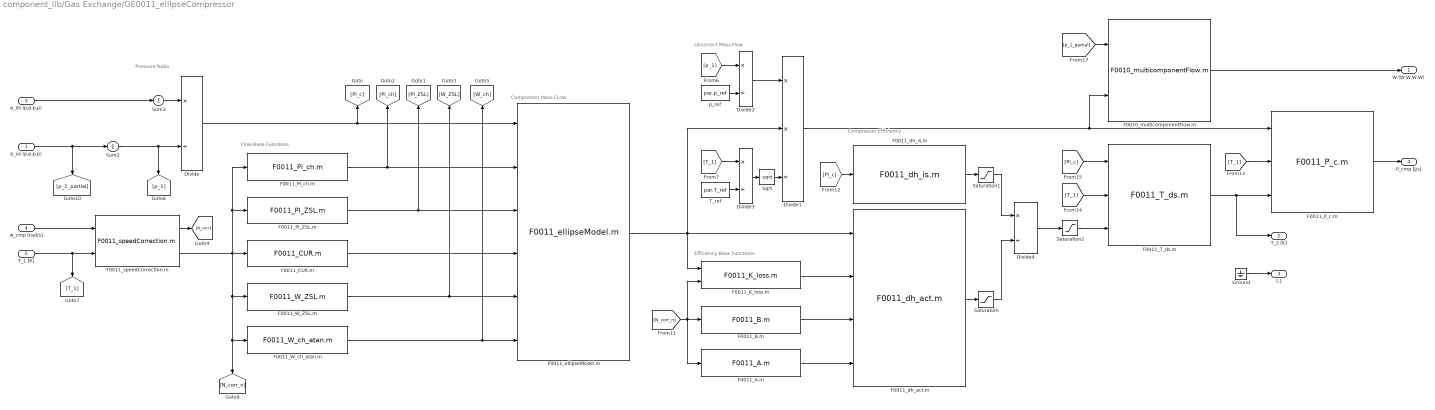
== system component_lib/Gas Exchange/GE0011_ellipseCompressor ==
  note: Compressor Mass FLow
  note: Compressor Efficiency
  note: Efficiency Base Functions
  note: Pressure Ratio
  note: Flow Base Functions
  note: Uncorrect Mass Flow
  p_us (p,p,p,p) : Inport
  T_1 [K] : Inport  Port=2
  p_ds (p,p,p,p) : Inport  Port=3
  w_cmp [rad/s] : Inport  Port=4
  Divide{,2..4} (4 alike) : Product  Inputs=*/
  Divide1 : Product  Inputs=**/
  F0010_multicomponentFlow.m : base_lib/F0010_gasFlow/F0010_multicomponentFlow.m  SystemSampleTime=-1  VariantActivationTime=update diagram  Latency=0  AutoFrameSizeCalculation=off
  F0011_A.m : base_lib/F0011_ellipseCompressor2/F0011_A.m  SystemSampleTime=-1  VariantActivationTime=update diagram  Latency=0  AutoFrameSizeCalculation=off
  F0011_B.m : base_lib/F0011_ellipseCompressor2/F0011_B.m  SystemSampleTime=-1  VariantActivationTime=update diagram  Latency=0  AutoFrameSizeCalculation=off
  F0011_CUR.m : base_lib/F0011_ellipseCompressor2/F0011_CUR.m  SystemSampleTime=-1  VariantActivationTime=update diagram  Latency=0  AutoFrameSizeCalculation=off
  F0011_K_loss.m : base_lib/F0011_ellipseCompressor2/F0011_K_loss.m  SystemSampleTime=-1  VariantActivationTime=update diagram  Latency=0  AutoFrameSizeCalculation=off
  F0011_PI_ZSL.m : base_lib/F0011_ellipseCompressor2/F0011_PI_ZSL.m  SystemSampleTime=-1  VariantActivationTime=update diagram  Latency=0  AutoFrameSizeCalculation=off
  F0011_P_c.m : base_lib/F0011_ellipseCompressor2/F0011_P_c.m  SystemSampleTime=-1  VariantActivationTime=update diagram  Latency=0  AutoFrameSizeCalculation=off
  F0011_Pi_ch.m : base_lib/F0011_ellipseCompressor2/F0011_Pi_ch.m  SystemSampleTime=-1  VariantActivationTime=update diagram  Latency=0  AutoFrameSizeCalculation=off
  F0011_T_ds.m : base_lib/F0011_ellipseCompressor2/F0011_T_ds.m  SystemSampleTime=-1  VariantActivationTime=update diagram  Latency=0  AutoFrameSizeCalculation=off
  F0011_W_ZSL.m : base_lib/F0011_ellipseCompressor2/F0011_W_ZSL.m  SystemSampleTime=-1  VariantActivationTime=update diagram  Latency=0  AutoFrameSizeCalculation=off
  F0011_W_ch_atan.m : base_lib/F0011_ellipseCompressor2/F0011_W_ch_atan.m  SystemSampleTime=-1  VariantActivationTime=update diagram  Latency=0  AutoFrameSizeCalculation=off
  F0011_dh_act.m : base_lib/F0011_ellipseCompressor2/F0011_dh_act.m  SystemSampleTime=-1  VariantActivationTime=update diagram  Latency=0  AutoFrameSizeCalculation=off
  F0011_dh_is.m : base_lib/F0011_ellipseCompressor2/F0011_dh_is.m  SystemSampleTime=-1  VariantActivationTime=update diagram  Latency=0  AutoFrameSizeCalculation=off
  F0011_ellipseModel.m : base_lib/F0011_ellipseCompressor2/F0011_ellipseModel.m  SystemSampleTime=-1  VariantActivationTime=update diagram  Latency=0  AutoFrameSizeCalculation=off
  F0011_speedCorrection.m : base_lib/F0011_ellipseCompressor2/F0011_speedCorrection.m  SystemSampleTime=-1  VariantActivationTime=update diagram  Latency=0  AutoFrameSizeCalculation=off
  Ground : Ground
  Saturation : Saturate  UpperLimit=inf  LowerLimit=1e-4
  Saturation1 : Saturate  UpperLimit=inf  LowerLimit=1e-4
  Saturation2 : Saturate  UpperLimit=1  LowerLimit=1e-3
  Sqrt : Sqrt  SaturateOnIntegerOverflow=on
  Sum2 : Sum  Inputs=|+|
  Sum3 : Sum  Inputs=|+|
  T_ref : Constant  Value=par.T_ref
  p_ref : Constant  Value=par.p_ref
  W (W,W,W,W) : Outport
  T_2 [K] : Outport  Port=2
  "[-]" : Outport  Port=3
  P_cmp [J/s] : Outport  Port=4
  wires:
  Sum3/1 -> Divide/1
  T_1 [K]/1 -> F0011_speedCorrection.m/2, [T_1]
  F0011_CUR.m/1 -> F0011_ellipseModel.m/4
  F0011_PI_ZSL.m/1 -> F0011_ellipseModel.m/3, [PI_ZSL]
  F0011_W_ZSL.m/1 -> F0011_ellipseModel.m/5, [W_ZSL]
  F0011_W_ch_atan.m/1 -> F0011_ellipseModel.m/6, [W_ch]
  F0011_speedCorrection.m/2 -> [N_corr_n], F0011_W_ch_atan.m/1, F0011_W_ZSL.m/1, F0011_Pi_ch.m/1, F0011_PI_ZSL.m/1, F0011_CUR.m/1
  Divide/1 -> F0011_ellipseModel.m/1, [Pi_c]
  F0011_speedCorrection.m/1 -> [N_corr]
  Divide1/1 -> F0010_multicomponentFlow.m/2, F0011_P_c.m/1
  p_ref/1 -> Divide2/2
  Divide2/1 -> Divide1/1
  [p_1] -> Divide2/1
  [T_1] -> Divide3/1
  T_ref/1 -> Divide3/2
  Divide3/1 -> Sqrt/1
  Sqrt/1 -> Divide1/3
  F0011_Pi_ch.m/1 -> F0011_ellipseModel.m/2, [Pi_ch]
  F0011_K_loss.m/1 -> F0011_dh_act.m/2
  F0011_B.m/1 -> F0011_dh_act.m/3
  F0011_A.m/1 -> F0011_dh_act.m/4
  [N_corr_n] -> F0011_K_loss.m/2, F0011_B.m/1, F0011_A.m/1
  [Pi_c] -> F0011_dh_is.m/1
  F0011_dh_act.m/1 -> Saturation/1
  F0011_dh_is.m/1 -> Saturation1/1
  Saturation1/1 -> Divide4/1
  Saturation/1 -> Divide4/2
  Divide4/1 -> Saturation2/1
  Saturation2/1 -> F0011_T_ds.m/3
  F0011_T_ds.m/1 -> T_2 [K]/1, F0011_P_c.m/3
  [T_1] -> F0011_P_c.m/2
  [T_1] -> F0011_T_ds.m/2
  [Pi_c] -> F0011_T_ds.m/1
  w_cmp [rad/s]/1 -> F0011_speedCorrection.m/1
  p_us (p,p,p,p)/1 -> Sum2/1, [p_1_partial]
  Sum2/1 -> Divide/2, [p_1]
  [p_1_partial] -> F0010_multicomponentFlow.m/1
  F0010_multicomponentFlow.m/1 -> W (W,W,W,W)/1
  F0011_ellipseModel.m/1 -> Divide1/2, F0011_K_loss.m/1, F0011_dh_act.m/1
  p_ds (p,p,p,p)/1 -> Sum3/1
  Ground/1 -> "[-]"/1
  F0011_P_c.m/1 -> P_cmp [J/s]/1

== system component_lib/Gas Exchange/GE0012_throttle ==
  p_1 [Pa] : Inport
  T_1 [K] : Inport  Port=2
  p_2 [Pa] : Inport  Port=3
  alpha [-] : Inport  Port=4
  F0008_throttleFlow2.m : base_lib/F0008_throttle/F0008_throttleFlow2.m  SystemSampleTime=-1  VariantActivationTime=update diagram  Latency=0  AutoFrameSizeCalculation=off
  Ground : Ground
  W [kg/s] : Outport
  T_2 [K] : Outport  Port=2
  "[--]" : Outport  Port=3
  "[---]" : Outport  Port=4
  wires:
  Ground/1 -> "[---]"/1, "[--]"/1
  F0008_throttleFlow2.m/1 -> W [kg/s]/1
  T_1 [K]/1 -> F0008_throttleFlow2.m/3, T_2 [K]/1, F0008_throttleFlow2.m/4
  alpha [-]/1 -> F0008_throttleFlow2.m/5
  p_1 [Pa]/1 -> F0008_throttleFlow2.m/1
  p_2 [Pa]/1 -> F0008_throttleFlow2.m/2

== system component_lib/Gas Exchange/GE0013_simpleEjector ==
  p_p [Pa] : Inport
  T_p [K] : Inport  Port=2
  p_s [Pa] : Inport  Port=3
  T_s [K] : Inport  Port=4
  p_b [Pa] : Inport  Port=5
  Divide : Product  Inputs=*/
  F0010_multicomponentFlow.m : base_lib/F0010_gasFlow/F0010_multicomponentFlow.m  SystemSampleTime=-1  VariantActivationTime=update diagram  Latency=0  AutoFrameSizeCalculation=off
  F0010_multicomponentFlow.m1 : base_lib/F0010_gasFlow/F0010_multicomponentFlow.m  SystemSampleTime=-1  VariantActivationTime=update diagram  Latency=0  AutoFrameSizeCalculation=off
  F0010_vaporSaturationPressure.m : base_lib/F0010_gasFlow/F0010_vaporSaturationPressure.m  SystemSampleTime=-1  VariantActivationTime=update diagram  Latency=0  AutoFrameSizeCalculation=off
  F0013_ejectorModel.m : base_lib/F0013_simpleEjector/F0013_ejectorModel.m  SystemSampleTime=-1  VariantActivationTime=update diagram  Latency=0  AutoFrameSizeCalculation=off
  Selector : Selector  InputPortWidth=4  IndexOptions=Index vector (dialog)  Indices=3  OutputSizes=1
  Sum : Sum  Inputs=+
  Sum1 : Sum  Inputs=+
  Sum2 : Sum  Inputs=+
  W_p [kg/s] : Outport
  W_s [kg/s] : Outport  Port=2
  phi [-] : Outport  Port=3
  w [-] : Outport  Port=4
  wires:
  p_p [Pa]/1 -> Sum/1, [P_p]
  Sum/1 -> F0013_ejectorModel.m/1
  p_s [Pa]/1 -> Sum1/1, [P_s]
  Sum1/1 -> F0013_ejectorModel.m/2
  Sum2/1 -> F0013_ejectorModel.m/3
  p_b [Pa]/1 -> Sum2/1
  F0013_ejectorModel.m/1 -> F0010_multicomponentFlow.m/2
  F0010_multicomponentFlow.m/1 -> W_p [kg/s]/1
  F0013_ejectorModel.m/2 -> F0010_multicomponentFlow.m1/2
  F0010_multicomponentFlow.m1/1 -> W_s [kg/s]/1
  [P_p] -> F0010_multicomponentFlow.m/1
  [P_s] -> F0010_multicomponentFlow.m1/1
  F0013_ejectorModel.m/3 -> phi [-]/1
  T_p [K]/1 -> [T_p], F0013_ejectorModel.m/4
  T_s [K]/1 -> [T_s], F0013_ejectorModel.m/5, F0010_vaporSaturationPressure.m/1
  [P_s] -> Selector/1
  Divide/1 -> F0013_ejectorModel.m/6
  Selector/1 -> Divide/1
  F0010_vaporSaturationPressure.m/1 -> Divide/2
  F0013_ejectorModel.m/4 -> w [-]/1

== system component_lib/Gas Exchange/GE0014_flowValve ==
  p_1 [Pa] : Inport
  T_1 [K] : Inport  Port=2
  p_2 [Pa] : Inport  Port=3
  T_2 [K] : Inport  Port=4
  open [-] : Inport  Port=5
  F0010_compressibleRestriction.m : base_lib/F0010_gasFlow/F0010_compressibleRestriction.m  SystemSampleTime=-1  VariantActivationTime=update diagram  Latency=0  AutoFrameSizeCalculation=off
      settings: SourceProductBaseCode=SL
  Ground : Ground
  W [kg/s] : Outport
  "[-]" : Outport  Port=2
  "[--]" : Outport  Port=3
  "[---]" : Outport  Port=4
  wires:
  p_1 [Pa]/1 -> F0010_compressibleRestriction.m/1
  p_2 [Pa]/1 -> F0010_compressibleRestriction.m/2
  T_1 [K]/1 -> F0010_compressibleRestriction.m/3
  Ground/1 -> "[-]"/1, "[--]"/1, "[---]"/1
  F0010_compressibleRestriction.m/1 -> W [kg/s]/1
  T_2 [K]/1 -> F0010_compressibleRestriction.m/4
  open [-]/1 -> F0010_compressibleRestriction.m/5

== system component_lib/Gas Exchange/GE0015_linearRestriction ==
  p_1 (p,p,p,p) : Inport
  p_2 (p,p,p,p) : Inport  Port=2
  F0010_linearFlowRestriction.m : base_lib/F0010_gasFlow/F0010_linearFlowRestriction.m  SystemSampleTime=-1  VariantActivationTime=update diagram  Latency=0  AutoFrameSizeCalculation=off
  W (W,W,W,W) : Outport
  wires:
  F0010_linearFlowRestriction.m/1 -> W (W,W,W,W)/1
  p_1 (p,p,p,p)/1 -> F0010_linearFlowRestriction.m/1
  p_2 (p,p,p,p)/1 -> F0010_linearFlowRestriction.m/2

== system component_lib/Mission/MN0001_profile ==
  v [m/s] : Inport
  Altitute lookup table : Lookup_n-D  NumberOfTableDimensions=1  BreakpointsForDimension1=ECCV_r.distance  Table=ECCV_r.altitude  InternalRulePriority=Speed  RndMeth=Simplest  InputSameDT=on
  Compare To Constant : simulink/Logic and Bit Operations/Compare To Constant  relop=>=  const=ECCV_r.distance(end)  OutDataTypeStr=boolean
  Constant1 : Constant  Value=ECCV_r.slope
  Find current index of distance vector : Lookup_n-D  NumberOfTableDimensions=1  BreakpointsForDimension1=ECCV_r.distance  Table=1:length(ECCV_r.distance)  InterpMethod=Nearest  InternalRulePriority=Speed  RndMeth=Simplest  InputSameDT=on
  Initial position : Constant  Value=x0
  Integrator1 : Integrator  InitialConditionSource=external
  Selector : Selector  InputPortWidth=length(ECCV_r.slope)  IndexOptions=Starting index (port)  Indices=[1 3]  OutputSizes=N_lookahead
  Slope lookup table : Lookup_n-D  NumberOfTableDimensions=1  BreakpointsForDimension1=ECCV_r.distance  Table=ECCV_r.slope  InternalRulePriority=Speed  RndMeth=Simplest  InputSameDT=on
  Stop Simulation : Stop
  slope [rad] : Outport
  altitude [m] : Outport  Port=2
  distance [m] : Outport  Port=3
  slope_lookahead [rad] : Outport  Port=4
  wires:
  Integrator1/1 -> Find current index of distance vector/1, Altitute lookup table/1, Slope lookup table/1, distance [m]/1, Compare To Constant/1
  Slope lookup table/1 -> slope [rad]/1
  Altitute lookup table/1 -> altitude [m]/1
  Compare To Constant/1 -> Stop Simulation/1
  Selector/1 -> slope_lookahead [rad]/1
  Constant1/1 -> Selector/1
  Find current index of distance vector/1 -> Selector/2
  Initial position/1 -> Integrator1/2
  v [m/s]/1 -> Integrator1/1

== system component_lib/Mission/MN0002_ambient ==
  note: 4 % per km decrease
  altitude [m] : Inport
  Constant : Constant  Value=RH_0
  F0018_troposphereModel.m : base_lib/F0018_ambientProperties/F0018_troposphereModel.m  SystemSampleTime=-1  VariantActivationTime=update diagram  Latency=0  AutoFrameSizeCalculation=off
      settings: SourceProductBaseCode=SL
  Gain : Gain  Gain=0.04e-3
  Product : Product
  Sum : Sum  Inputs=|+-
  T [K] : Outport
  p [Pa] : Outport  Port=2
  RH [-] : Outport  Port=3
  wires:
  F0018_troposphereModel.m/2 -> T [K]/1
  F0018_troposphereModel.m/1 -> p [Pa]/1
  altitude [m]/1 -> Gain/1, F0018_troposphereModel.m/1
  Gain/1 -> Product/2
  Constant/1 -> Sum/1, Product/1
  Product/1 -> Sum/2
  Sum/1 -> RH [-]/1

== system component_lib/Powertrain/PT0001_simpleVehicle ==
  note: Tractive force
  Tq_in [Nm] : Inport
  alpha [rad] : Inport  Port=2
  brake [-] : Inport  Port=3
  Abs : Abs
  Abs1 : Abs
  Constant : Constant  Value=par.r_w
  Divide : Product  Inputs=*/
  Divide1 : Product  Inputs=*/
  F0006_airDrag.m : base_lib/F0006_truckBenchmark/F0006_airDrag.m  SystemSampleTime=-1  VariantActivationTime=update diagram  Latency=0  AutoFrameSizeCalculation=off
  F0006_brakeForce.m : base_lib/F0006_truckBenchmark/F0006_brakeForce.m  SystemSampleTime=-1  VariantActivationTime=update diagram  Latency=0  AutoFrameSizeCalculation=off
  F0006_gravitationalForce.m : base_lib/F0006_truckBenchmark/F0006_gravitationalForce.m  SystemSampleTime=-1  VariantActivationTime=update diagram  Latency=0  AutoFrameSizeCalculation=off
  F0006_rollingResistance.m : base_lib/F0006_truckBenchmark/F0006_rollingResistance.m  SystemSampleTime=-1  VariantActivationTime=update diagram  Latency=0  AutoFrameSizeCalculation=off
  Gain : Gain  Gain=1/par.m
  Initial speed : Constant  Value=par.v0
  Integrator2 : Integrator  InitialConditionSource=external
  Sum : Sum  Inputs=+++
  Sum1 : Sum  Inputs=|+-
  Sum2 : Sum  Inputs=++|
  v [m/s] : Outport
  w_w [rad/s] : Outport  Port=2
  wires:
  alpha [rad]/1 -> F0006_gravitationalForce.m/1, F0006_rollingResistance.m/2
  Initial speed/1 -> Integrator2/2
  F0006_airDrag.m/1 -> Sum/1
  F0006_rollingResistance.m/1 -> Sum/2
  Sum1/1 -> Gain/1
  F0006_gravitationalForce.m/1 -> Sum/3
  Gain/1 -> Integrator2/1
  Sum2/1 -> Sum1/2
  Sum/1 -> Sum2/2
  Integrator2/1 -> Divide1/1, Abs1/1, Abs/1, v [m/s]/1
  Abs/1 -> F0006_airDrag.m/1
  Abs1/1 -> F0006_rollingResistance.m/1
  Divide1/1 -> w_w [rad/s]/1
  brake [-]/1 -> F0006_brakeForce.m/1
  F0006_brakeForce.m/1 -> Sum2/1
  Divide/1 -> Sum1/1
  Tq_in [Nm]/1 -> Divide/1
  Constant/1 -> Divide1/2, Divide/2

== system component_lib/Powertrain/PT0002_simpleMotor ==
  Tq_ref [Nm] : Inport
  V [V] : Inport  Port=2
  w_em [rad/s] : Inport  Port=3
  F0009_currentDemand.m : base_lib/F0009_simpleTractionMotor/F0009_currentDemand.m  SystemSampleTime=-1  VariantActivationTime=update diagram  Latency=0  AutoFrameSizeCalculation=off
      settings: SourceProductBaseCode=SL
  Torque dynamics : TransferFcn  Denominator=[T_s 1]
  Tq_em [Nm] : Outport
  I_em [A] : Outport  Port=2
  Q_gen [J/s] : Outport  Port=3
  wires:
  w_em [rad/s]/1 -> F0009_currentDemand.m/3
  V [V]/1 -> F0009_currentDemand.m/2
  Torque dynamics/1 -> Tq_em [Nm]/1, F0009_currentDemand.m/1
  Tq_ref [Nm]/1 -> Torque dynamics/1
  F0009_currentDemand.m/2 -> I_em [A]/1
  F0009_currentDemand.m/1 -> Q_gen [J/s]/1

== system component_lib/Powertrain/PT0003_gearBox ==
  Tq_in [Nm] : Inport
  w_out [rad/s] : Inport  Port=2
  gear  [-] : Inport  Port=3
  clutch  [-] : Inport  Port=4
  1-D Lookup Table : Lookup_n-D  NumberOfTableDimensions=1  BreakpointsForDimension1=par.gears  Table=par.gear_ratios  InterpMethod=Nearest  InternalRulePriority=Speed  RndMeth=Simplest  InputSameDT=on
  F0006_gearBox.m : base_lib/F0006_truckBenchmark/F0006_gearBox.m  SystemSampleTime=-1  VariantActivationTime=update diagram  Latency=0  AutoFrameSizeCalculation=off
      settings: SourceProductBaseCode=SL
  Product : Product
  Tq_out [Nm] : Outport
  w_in [rad/s] : Outport  Port=2
  wires:
  w_out [rad/s]/1 -> F0006_gearBox.m/2
  Tq_in [Nm]/1 -> F0006_gearBox.m/1
  F0006_gearBox.m/2 -> w_in [rad/s]/1
  1-D Lookup Table/1 -> F0006_gearBox.m/3
  gear  [-]/1 -> 1-D Lookup Table/1
  clutch  [-]/1 -> Product/1
  F0006_gearBox.m/1 -> Product/2
  Product/1 -> Tq_out [Nm]/1
